simulink model "FFW"  (R2022b)
settings: Solver=VariableStepAuto  StartTime=0.0  StopTime=10.0  RelTol=1e-3
settings Model: Creator=emanuelevitetta  LastModifiedBy=emanuelevitetta

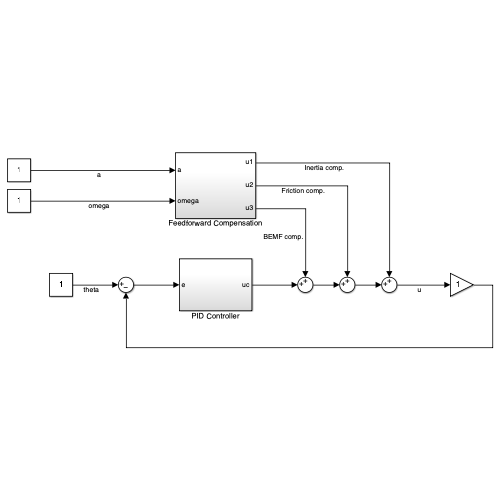
[thumbnail: Simulink's stored preview of the top-level diagram]
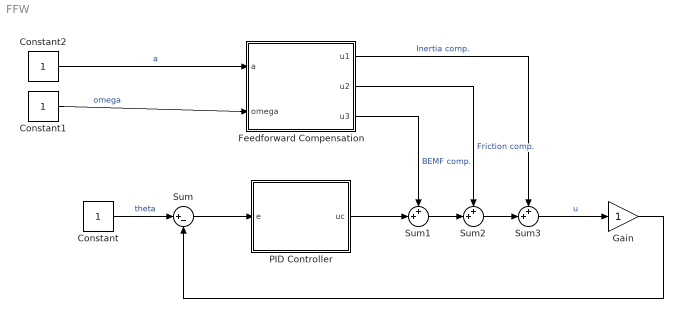
== system FFW ==
  Constant : Constant
  Constant1 : Constant
  Constant2 : Constant
  Feedforward Compensation : Subsystem
  Gain : Gain
  PID Controller : Subsystem
  Sum : Sum  Inputs=|+-
  Sum1 : Sum  Inputs=++|
  Sum2 : Sum  Inputs=++|
  Sum3 : Sum  Inputs=++|
  wires:
  Constant/1 -> Sum/1  "theta"
  Sum/1 -> PID Controller/1(e)
  Gain/1 -> Sum/2
  PID Controller/1(uc) -> Sum1/2
  Sum1/1 -> Sum2/2
  Sum2/1 -> Sum3/2
  Sum3/1 -> Gain/1  "u"
  Constant2/1 -> Feedforward Compensation/1(a)  "a"
  Constant1/1 -> Feedforward Compensation/2(omega)  "omega"
  Feedforward Compensation/1(u1) -> Sum3/1  "Inertia comp."
  Feedforward Compensation/2(u2) -> Sum2/1  "Friction comp."
  Feedforward Compensation/3(u3) -> Sum1/1  "BEMF comp."

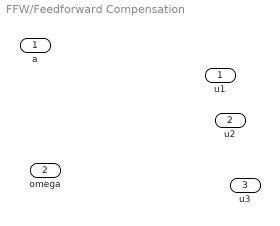
== system FFW/Feedforward Compensation ==
  a : Inport
  omega : Inport  Port=2
  u1 : Outport
  u2 : Outport  Port=2
  u3 : Outport  Port=3

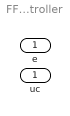
== system FFW/PID Controller ==
  e : Inport
  uc : Outport
